simulink model "simulation_ex_5"  (R2021a)
settings: Solver=VariableStepAuto  StartTime=0.0  StopTime=10000  RelTol=1e-3
settings Model: Creator=HanO  LastModifiedBy=HanO

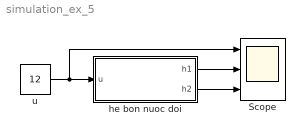
== system simulation_ex_5 ==
  Scope : Scope  NumInputPorts=3
  he bon nuoc doi : Subsystem  mask{AA1=10, AA2=15, k=0.5, a1=0.5, a2=0.2, cd1=0.4, cd2=0.6, g=9.81, h1_zero=0, h2_zero=0}
      mask prompts: AA1 "Tiết diện ngang bồn 1"; AA2 "Tiết diện ngang bồn 2"; k "Hệ số công suất máy bơm"; a1 "Tiết diện valve xả bồn 1"; a2 "Tiết diện valve xả bồn 2"; cd1 "Hệ số xả valve bồn 1"; cd2 "Hệ số xả valve bồn 2"; g "Gia tốc trọng trường"; h1_zero "Chiều cao mực nước bồn 1 ban đầu"; h2_zero "Chiều cao mực nước bồn 2 ban đầu"
  u : Constant  Value=12
  wires:
  u/1 -> Scope/1, he bon nuoc doi/1(u)
  he bon nuoc doi/1(h1) -> Scope/2
  he bon nuoc doi/2(h2) -> Scope/3

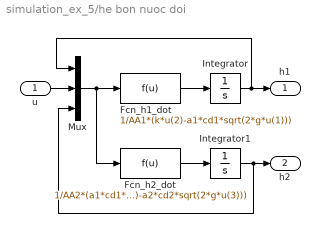
== system simulation_ex_5/he bon nuoc doi ==
  u : Inport
  Fcn_h1_dot : Fcn  Expr=1/AA1*(k*u(2)-a1*cd1*sqrt(2*g*u(1)))
  Fcn_h2_dot : Fcn  Expr=1/AA2*(a1*cd1*sqrt(2*g*u(1))-a2*cd2*sqrt(2*g*u(3)))
  Integrator : Integrator  InitialCondition=h1_zero
  Integrator1 : Integrator  InitialCondition=h2_zero
  Mux : Mux  Inputs=3
  h1 : Outport
  h2 : Outport  Port=2
  wires:
  Fcn_h1_dot/1 -> Integrator/1
  Fcn_h2_dot/1 -> Integrator1/1
  u/1 -> Mux/2
  Mux/1 -> Fcn_h2_dot/1, Fcn_h1_dot/1
  Integrator/1 -> Mux/1, h1/1
  Integrator1/1 -> h2/1, Mux/3
